simulink model "dfilter_3stage_start"  (Simulink 8.4)
settings: Solver=ode45  StartTime=0.0  StopTime=10.0  RelTol=1e-3
libraries: simulink_extras x1, simulink x1
settings Model: Creator=amatsumo  LastModifiedBy=kotsuka
settings DataIOCC: SaveOutput=off  SignalLogging=off  SaveTime=off
settings OptimizationCC: BlockReduction=off  ConditionallyExecuteInputs=off  InlineParams=on
settings DebuggingCC: AlgebraicLoopMsg=error  SingleTaskRateTransMsg=error  FcnCallInpInsideContextMsg=EnableAllAsWarning
settings HardwareCC: ProdHWDeviceType=ASIC/FPGA->ASIC/FPGA  TargetLongLongMode=on  TargetIntDivRoundTo=Zero  TargetEndianess=LittleEndian  TargetHWDeviceType=MATLAB Host  ProdEqTarget=off

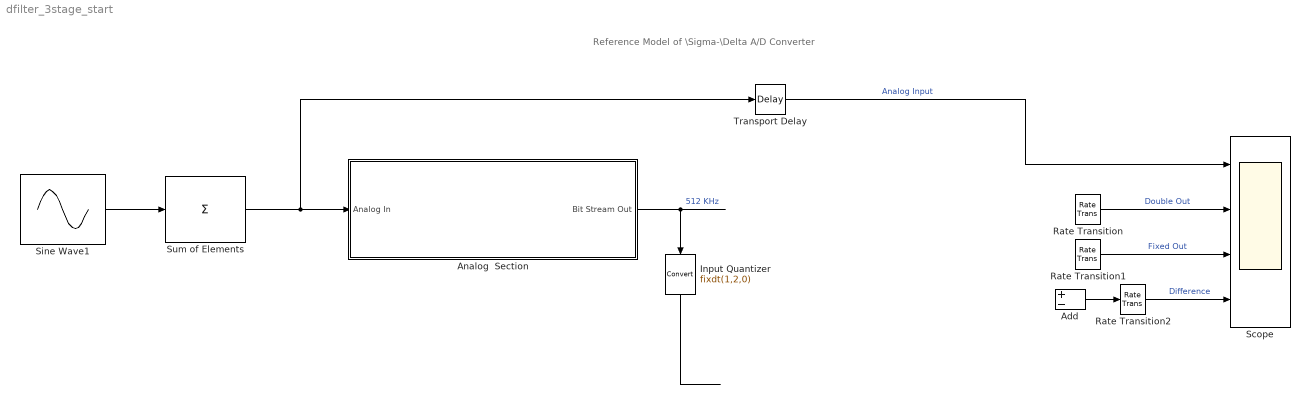
== system dfilter_3stage_start ==
  note: Reference Model of
      | \Sigma-\Delta A/D Converter
  Add : Sum  Inputs=+-
  Analog  Section : Subsystem
  Input Quantizer : DataTypeConversion  OutDataTypeStr=fixdt(1,2,0)  RndMeth=Round  SaturateOnIntegerOverflow=on
  Rate Transition : RateTransition
  Rate Transition1 : RateTransition
  Rate Transition2 : RateTransition
  Scope : Scope  NumInputPorts=4
      settings: TimeRange=0.0175  YMin=-1~-1~-0.75~-0.4  YMax=1~1~1~0.4
  Sine Wave1 : Sin  Amplitude=0.5  Frequency=2*pi*[1500 1750]  SampleTime=0
  Sum of Elements : Sum  Inputs=+
  Transport Delay : TransportDelay  DelayTime=(1/512e3*(31/2))+(8/512e3*(7/2))+(16/512e3*(121/2))
  wires:
  Analog  Section/1(Bit Stream Out) -> Input Quantizer/1  "512 KHz"
  ? -> Add/1, Rate Transition/1  "Digital Output 8 KHz"
  Sum of Elements/1 -> Transport Delay/1, Analog  Section/1(Analog In)
  Sine Wave1/1 -> Sum of Elements/1
  Transport Delay/1 -> Scope/1  "Analog Input"
  ? -> Add/2, Rate Transition1/1
  Add/1 -> Rate Transition2/1
  Input Quantizer/1 -> ?
  Rate Transition/1 -> Scope/2  "Double Out"
  Rate Transition1/1 -> Scope/3  "Fixed Out"
  Rate Transition2/1 -> Scope/4  "Difference"

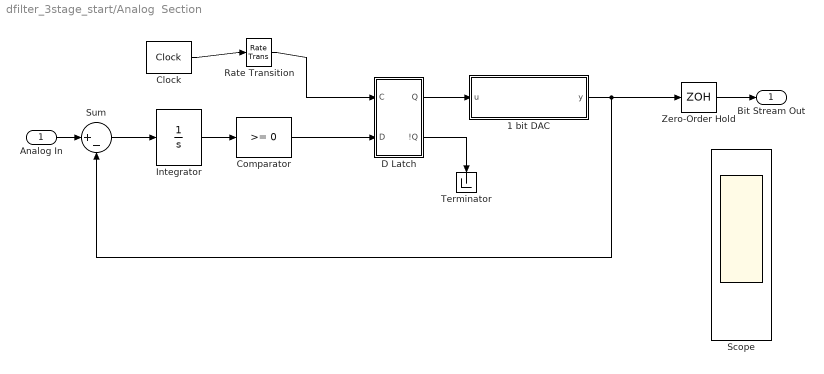
== system dfilter_3stage_start/Analog  Section ==
  Analog In : Inport
  1 bit DAC : MATLAB Function  TreatAsAtomicUnit=on
  Clock : simulink_extras/Flip Flops/Clock  period=1/512000
  Comparator : simulink/Logic and Bit Operations/Compare To Zero  relop=>=  OutDataTypeStr=boolean  ZeroCross=off
  D Latch : Subsystem  AncestorBlock=simulink_extras/Flip Flops/D Latch  mask(DLatch){}
      mask help: D Latch Flip-Flop Block
      mask Help:
      | The D latch flip-flop block has the following characteristic table:
      | <pre>
      |   Q(t)  D(t)     Q(tnext)
      |   ------------------------
      |    0      0       0
      |    0      1       1
      |    1      0       0
      |    1      1       1
      | </pre>
      | The D latch transfers "data" into a memory element (flip-flop).  The D latch
      | flip-flop is sometimes called a gated D-latch. The chip enable input signal, C,
      | is sometimes given the designation G (for gate) to indicate that this input
      | enables the gated latch allowing data entry into the flip-flop.
  Integrator : Integrator
  Rate Transition : RateTransition
  Scope : Scope  NumInputPorts=4
      settings: TimeRange=0.0175  YMin=-1~-1~-0.75~-0.4  YMax=1~1~1~0.4
  Sum : Sum  Inputs=|+-
  Terminator : Terminator
  Zero-Order Hold : ZeroOrderHold  SampleTime=1/512000
  Bit Stream Out : Outport
  wires:
  Sum/1 -> Integrator/1
  Integrator/1 -> Comparator/1
  D Latch/1(Q) -> 1 bit DAC/1(u)
  Comparator/1 -> D Latch/2(D)
  Clock/1 -> Rate Transition/1
  Analog In/1 -> Sum/1
  D Latch/2(!Q) -> Terminator/1
  1 bit DAC/1(y) -> Sum/2, Zero-Order Hold/1
  Zero-Order Hold/1 -> Bit Stream Out/1
  Rate Transition/1 -> D Latch/1(C)

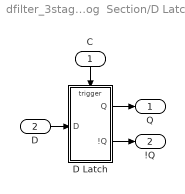
== system dfilter_3stage_start/Analog  Section/D Latch ==
  C : Inport
  D : Inport  Port=2
  D Latch : Subsystem  TreatAsAtomicUnit=on
  Q : Outport
  !Q : Outport  Port=2  InitialOutput=1
  wires:
  C/1 -> D Latch/Trigger
  D Latch/1(Q) -> Q/1
  D/1 -> D Latch/1(D)
  D Latch/2(!Q) -> !Q/1

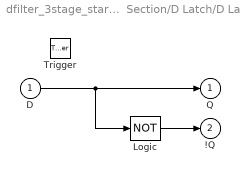
== system dfilter_3stage_start/Analog  Section/D Latch/D Latch ==
  D : Inport
  Trigger : TriggerPort  StatesWhenEnabling=reset
  Logic : Logic  Operator=NOT  Inputs=1
  Q : Outport  InitialOutput=0
  !Q : Outport  Port=2  InitialOutput=1
  wires:
  Logic/1 -> !Q/1
  D/1 -> Q/1, Logic/1

== matlab function Analog Section/1 bit DAC ==
  data: u input double; y output double
function y = DAC_1_bit(u)
% This block supports an embeddable subset of the MATLAB language.
% See the help menu for details.

% This code converts boolean input to a bipolar output (double precision). 

y=-1+2*u;
